simulink model "E_ZH_Z3"  (R2025a)
settings: Solver=VariableStepAuto  StartTime=0.0  StopTime=10.0  RelTol=1e-3
libraries: simulink x1, ZH_Z x1
settings Model: Creator=Szalay  LastModifiedBy=Szalay
settings RTWCC: RTWVerbose=off

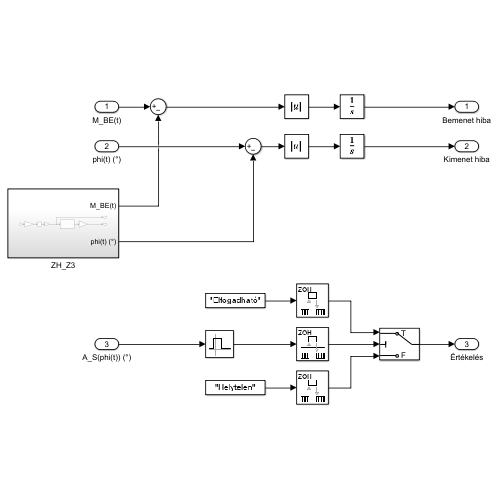
[thumbnail: Simulink's stored preview of the top-level diagram]
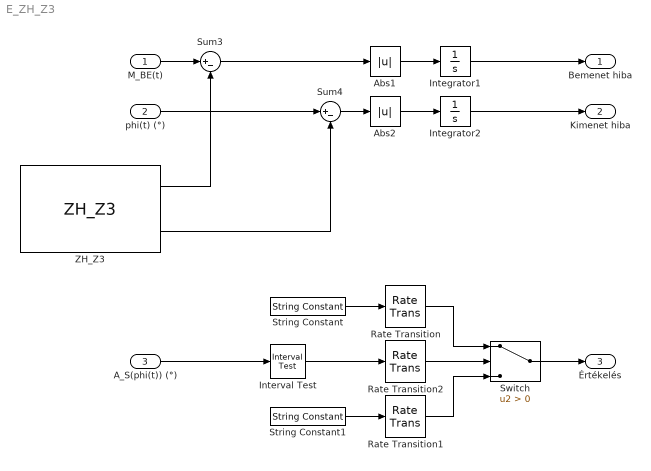
== system E_ZH_Z3 ==
  M_BE(t) : Inport  OutDataTypeStr=double  PortDimensions=1
  phi(t) (°) : Inport  Port=2  OutDataTypeStr=double  PortDimensions=1
  A_S(phi(t)) (°) : Inport  Port=3  OutDataTypeStr=double  PortDimensions=1
  Abs1 : Abs  SaturateOnIntegerOverflow=off
  Abs2 : Abs  SaturateOnIntegerOverflow=off
  Integrator1 : Integrator
  Integrator2 : Integrator
  Interval Test : simulink/Logic and Bit Operations/Interval Test  IntervalClosedRight=on  uplimit=109.5  IntervalClosedLeft=on  lowlimit=108.5  OutDataTypeStr=boolean
  Rate Transition : RateTransition  OutPortSampleTime=100e-3
  Rate Transition1 : RateTransition  OutPortSampleTime=100e-3
  Rate Transition2 : RateTransition  OutPortSampleTime=100e-3
  String Constant : StringConstant  String="\"Elfogadható\""
  String Constant1 : StringConstant  String="\"Helytelen\""
  Sum3 : Sum  Inputs=|+-
  Sum4 : Sum  Inputs=|+-
  Switch : Switch  Criteria=u2 > Threshold  SaturateOnIntegerOverflow=off  InputSameDT=off
  ZH_Z3 : ZH_Z/ZH_Z3  SystemSampleTime=-1  VariantActivationTime=update diagram  EmptyChoice=off  PassThrough=off  PassThroughVariantControl=(default)  EmptyChoiceVariantControl=(default)  AllowFlexibleInterface=on  Latency=0  AutoFrameSizeCalculation=off
  Bemenet hiba : Outport  OutDataTypeStr=double  PortDimensions=1  SampleTime=0
  Kimenet hiba : Outport  Port=2  OutDataTypeStr=double  PortDimensions=1  SampleTime=0
  Értékelés : Outport  Port=3  OutDataTypeStr=string  PortDimensions=1
  wires:
  Integrator1/1 -> Bemenet hiba/1
  M_BE(t)/1 -> Sum3/1
  Abs2/1 -> Integrator2/1
  Integrator2/1 -> Kimenet hiba/1
  Sum3/1 -> Abs1/1
  ZH_Z3/2 -> Sum4/2
  Sum4/1 -> Abs2/1
  ZH_Z3/1 -> Sum3/2
  phi(t) (°)/1 -> Sum4/1
  Abs1/1 -> Integrator1/1
  Switch/1 -> Értékelés/1
  String Constant/1 -> Rate Transition/1
  Rate Transition1/1 -> Switch/3
  A_S(phi(t)) (°)/1 -> Interval Test/1
  Rate Transition/1 -> Switch/1
  String Constant1/1 -> Rate Transition1/1
  Rate Transition2/1 -> Switch/2
  Interval Test/1 -> Rate Transition2/1
